simulink model "Control_PID_ISA"  (Simulink 7.8)
settings: Solver=ode45  StartTime=0  StopTime=30  FixedStep=0.05  MinStep=0.0001  RelTol=1e-6
values from neighbouring files (symbols this model uses):
  Kc = n(2)/d(2)    [pid2isa.m]
  Td = n(1)/n(2)    [pid2isa.m]
  Ti = n(2)/n(3)    [pid2isa.m]
undefined symbols (not defined in the file or in its folder): u10, u20
libraries: cstblocks x2
settings Model: Creator=sergarro  LastModifiedBy=sergarro
settings DebuggingCC: FcnCallInpInsideContextMsg=Use local settings  StrictBusMsg=Warning
settings SFSimCC: SimParseCustomCode=off

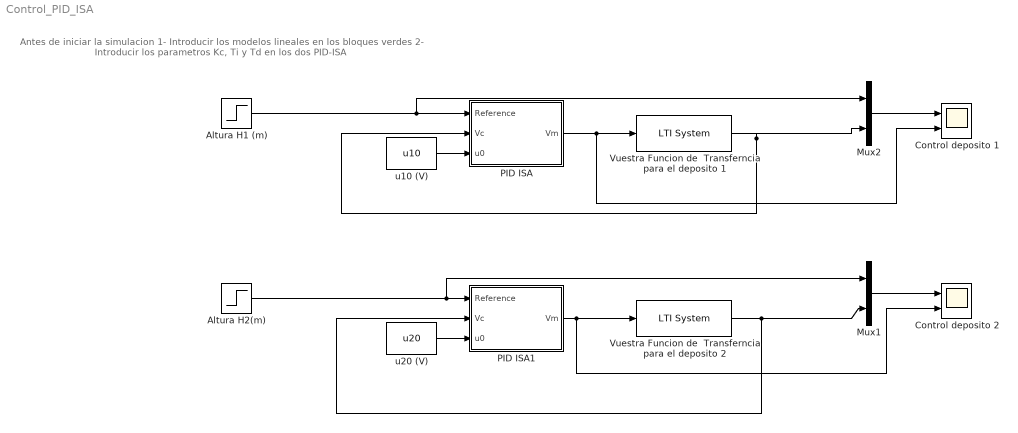
== system Control_PID_ISA ==
  note: Antes de iniciar la simulacion
      | 1- Introducir los modelos lineales en los bloques verdes
      | 2- Introducir los parametros Kc, Ti y Td en los dos PID-ISA
  Altura H1 (m) : Step  After=5  SampleTime=0.06
  Altura H2(m) : Step  After=5  SampleTime=0.06
  Control deposito 1 : Scope  NumInputPorts=2
      settings: TimeRange=30  YMin=-15~0  YMax=20~14  MaxDataPoints=100000
  Control deposito 2 : Scope  NumInputPorts=2
      settings: TimeRange=30  YMin=-15~0  YMax=20~14  SaveName=ScopeData2  MaxDataPoints=100000
  Mux1 : Mux  Inputs=2
  Mux2 : Mux  Inputs=2
  PID ISA : Subsystem  mask{kc=Kc, Ti=Ti, Td=Td}
  PID ISA1 : Subsystem  mask{kc=Kc, Ti=Ti, Td=Td}
  Vuestra Funcion de  Transferncia para el deposito 1 : cstblocks/LTI System  sys=Gx  IC=[]
  Vuestra Funcion de  Transferncia para el deposito 2 : cstblocks/LTI System  sys=Gy  IC=[]
  "u10 (V)   " : Constant  Value=u10
  u20 (V) : Constant  Value=u20
  wires:
  Altura H1 (m)/1 -> PID ISA/1(Reference), Mux2/1
  Vuestra Funcion de  Transferncia para el deposito 1/1 -> PID ISA/2(Vc), Mux2/2
  Vuestra Funcion de  Transferncia para el deposito 2/1 -> PID ISA1/2(Vc), Mux1/2
  Altura H2(m)/1 -> PID ISA1/1(Reference), Mux1/1
  "u10 (V)   "/1 -> PID ISA/3(u0)
  PID ISA/1(Vm) -> Vuestra Funcion de  Transferncia para el deposito 1/1, Control deposito 1/2
  PID ISA1/1(Vm) -> Vuestra Funcion de  Transferncia para el deposito 2/1, Control deposito 2/2
  u20 (V)/1 -> PID ISA1/3(u0)
  Mux1/1 -> Control deposito 2/1
  Mux2/1 -> Control deposito 1/1

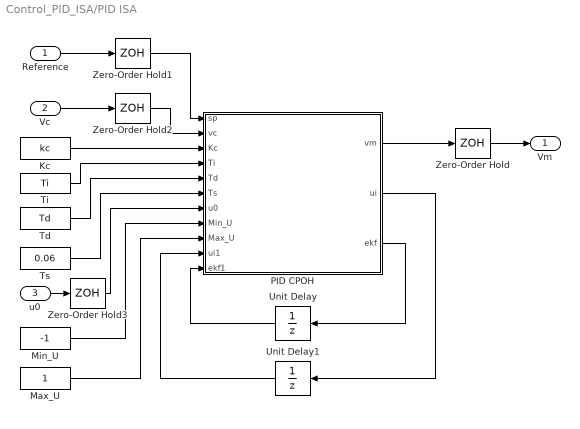
== system Control_PID_ISA/PID ISA ==
  Reference : Inport
  Vc : Inport  Port=2
  u0 : Inport  Port=3
  Kc : Constant  Value=kc
  Max_U : Constant
  Min_U : Constant  Value=-1
  PID CPOH : MATLAB Function  TreatAsAtomicUnit=on
  Td : Constant  Value=Td
  Ti : Constant  Value=Ti
  Ts : Constant  Value=0.06
  Unit Delay : UnitDelay  SampleTime=0.04
  Unit Delay1 : UnitDelay  SampleTime=0.04
  Zero-Order Hold{,1..3} (4 alike) : ZeroOrderHold  SampleTime=0.04
  Vm : Outport
  wires:
  Kc/1 -> PID CPOH/3(Kc)
  Ti/1 -> PID CPOH/4(Ti)
  Td/1 -> PID CPOH/5(Td)
  Ts/1 -> PID CPOH/6(Ts)
  u0/1 -> Zero-Order Hold3/1
  Min_U/1 -> PID CPOH/8(Min_U)
  Max_U/1 -> PID CPOH/9(Max_U)
  Unit Delay/1 -> PID CPOH/11(ekf1)
  PID CPOH/3(ekf) -> Unit Delay/1
  Unit Delay1/1 -> PID CPOH/10(ui1)
  PID CPOH/2(ui) -> Unit Delay1/1
  Reference/1 -> Zero-Order Hold1/1
  Vc/1 -> Zero-Order Hold2/1
  PID CPOH/1(vm) -> Zero-Order Hold/1
  Zero-Order Hold/1 -> Vm/1
  Zero-Order Hold1/1 -> PID CPOH/1(sp)
  Zero-Order Hold3/1 -> PID CPOH/7(u0)
  Zero-Order Hold2/1 -> PID CPOH/2(vc)

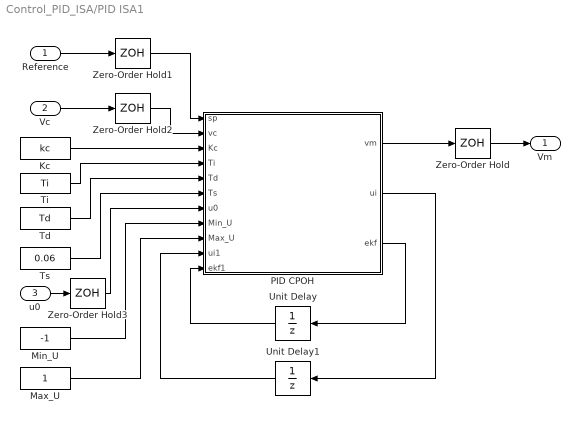
== system Control_PID_ISA/PID ISA1 ==
  Reference : Inport
  Vc : Inport  Port=2
  u0 : Inport  Port=3
  Kc : Constant  Value=kc
  Max_U : Constant
  Min_U : Constant  Value=-1
  PID CPOH : MATLAB Function  TreatAsAtomicUnit=on
  Td : Constant  Value=Td
  Ti : Constant  Value=Ti
  Ts : Constant  Value=0.06
  Unit Delay : UnitDelay  SampleTime=0.04
  Unit Delay1 : UnitDelay  SampleTime=0.04
  Zero-Order Hold{,1..3} (4 alike) : ZeroOrderHold  SampleTime=0.04
  Vm : Outport
  wires:
  Kc/1 -> PID CPOH/3(Kc)
  Ti/1 -> PID CPOH/4(Ti)
  Td/1 -> PID CPOH/5(Td)
  Ts/1 -> PID CPOH/6(Ts)
  u0/1 -> Zero-Order Hold3/1
  Min_U/1 -> PID CPOH/8(Min_U)
  Max_U/1 -> PID CPOH/9(Max_U)
  Unit Delay/1 -> PID CPOH/11(ekf1)
  PID CPOH/3(ekf) -> Unit Delay/1
  Unit Delay1/1 -> PID CPOH/10(ui1)
  PID CPOH/2(ui) -> Unit Delay1/1
  Reference/1 -> Zero-Order Hold1/1
  Vc/1 -> Zero-Order Hold2/1
  PID CPOH/1(vm) -> Zero-Order Hold/1
  Zero-Order Hold/1 -> Vm/1
  Zero-Order Hold1/1 -> PID CPOH/1(sp)
  Zero-Order Hold3/1 -> PID CPOH/7(u0)
  Zero-Order Hold2/1 -> PID CPOH/2(vc)

== matlab function PID ISA1/PID CPOH ==
  data: sp input double; vm output double; vc input double; Kc input double; Ti input double; Td input double; Ts input double; u0 input double; Min_U input double; Max_U input double; ui1 input double; ekf1 input double; ui output double; ekf output double
function [vm,ui,ekf] = fcn(sp,vc,Kc,Ti,Td,Ts,u0,Min_U,Max_U,ui1,ekf1)
%#codegen
% Variables auxiliares...
N =0; % N=0 desconecta el filtro de la derivada
b  = 1;      % Ponderacin de la ref en la accin Proporcional
c  = 1;      % Ponderacin de la ref en la accin derivada
offset = u0;  % offset, incluye el efecto de los puntos de
ki = 0;

if (Ti~=0)
    ki = (Kc*Ts)/Ti;
end

kd = (Kc*Td)/Ts;

if N~=0
    kn =Td/(N*Ts);
end

tauf = 0;
kf = tauf/Ts;

% Filtrado de la medida
if tauf == 0
    ykf=vc;
else
    ykf=(kf*ykf1+vc)/(kf+1);
end

% clculo termino proporcional...
% con ponderacion de la referencia...
up=Kc*(b*sp-ykf);

% clculo del termino derivada...
% con ponderacion de la referencia...
% y filtrado...

if (Td==0)
    ud=0;
    ekf=0;
else
    ek=c*sp-ykf;
    if N==0
        ekf=ek;
    else
        ekf=(kn*ekf1+ek)/(kn+1);
    end
    ud=kd*(ekf-ekf1);
end

% clculo termino integral...
if (Ti==0)
    ui=0;
else
    ui=ui1+ki*(sp-ykf);
end
vm = up+ui+ud+offset;

% Antiwindup...
% saturacin del incremento minimo (El incremento mnimo es de 0.005 mm)
% saturacin de la accin de control.
if (vm < Min_U)
    ui=ui1;
    vm=Min_U;
end
if (vm > Max_U)
    ui=ui1;
    vm= Max_U;
end

== matlab function PID ISA/PID CPOH ==
  data: sp input double; vm output double; vc input double; Kc input double; Ti input double; Td input double; Ts input double; u0 input double; Min_U input double; Max_U input double; ui1 input double; ekf1 input double; ui output double; ekf output double
function [vm,ui,ekf] = fcn(sp,vc,Kc,Ti,Td,Ts,u0,Min_U,Max_U,ui1,ekf1)
%#codegen
% Variables auxiliares...
N =0; % N=0 desconecta el filtro de la derivada
b  = 1;      % Ponderacin de la ref en la accin Proporcional
c  = 1;      % Ponderacin de la ref en la accin derivada
offset = u0;  % offset, incluye el efecto de los puntos de
ki = 0;

if (Ti~=0)
    ki = (Kc*Ts)/Ti;
end

kd = (Kc*Td)/Ts;

if N~=0
    kn =Td/(N*Ts);
end

tauf = 0;
kf = tauf/Ts;

% Filtrado de la medida
if tauf == 0
    ykf=vc;
else
    ykf=(kf*ykf1+vc)/(kf+1);
end

% clculo termino proporcional...
% con ponderacion de la referencia...
up=Kc*(b*sp-ykf);

% clculo del termino derivada...
% con ponderacion de la referencia...
% y filtrado...

if (Td==0)
    ud=0;
    ekf=0;
else
    ek=c*sp-ykf;
    if N==0
        ekf=ek;
    else
        ekf=(kn*ekf1+ek)/(kn+1);
    end
    ud=kd*(ekf-ekf1);
end

% clculo termino integral...
if (Ti==0)
    ui=0;
else
    ui=ui1+ki*(sp-ykf);
end
vm = up+ui+ud+offset;

% Antiwindup...
% saturacin del incremento minimo (El incremento mnimo es de 0.005 mm)
% saturacin de la accin de control.
if (vm < Min_U)
    ui=ui1;
    vm=Min_U;
end
if (vm > Max_U)
    ui=ui1;
    vm= Max_U;
end
